simulink model "Adaptive_Cruise_Contro_Final_KD_JB_TV_22"  (R2020a)
settings: Solver=FixedStepAuto  StartTime=0.0  StopTime=10.0  RelTol=1e-3  EnableMultiTasking=on
libraries: arduinolib x14, arduinosensorlib x1
settings Model: SILPILModeSetting=veronly  ExtModeTrigDuration=2  Creator=anuru  LastModifiedBy=anuru
settings OptimizationCC: EnhancedBackFolding=on  PassReuseOutputArgsAs=Individual arguments  ZeroExternalMemoryAtStartup=off  ZeroInternalMemoryAtStartup=off  MaxStackSize=64  OptimizeBlockOrder=speed  DifferentSizesBufferReuse=on  OptimizationCustomize=off  EfficientTunableParamExpr=on
settings DebuggingCC: ParameterTunabilityLossMsg=error
settings HardwareCC: ProdBitPerInt=16  ProdBitPerPointer=16  ProdBitPerSizeT=16  ProdBitPerPtrDiffT=16  ProdLargestAtomicFloat=None  ProdWordSize=8  ProdHWDeviceType=Atmel->AVR
settings SFSimCC: MATLABDynamicMemAlloc=off
settings RTWCC: SystemTargetFile=ert.tlc  HardwareBoard=Arduino Uno  TLCOptions=-aInlineSetEventsForThisBaseRateFcn=TLC_FALSE -aSuppressMultiTaskScheduler=TLC_FALSE -aRateBasedStepFcn=1  TemplateMakefile=ert_default_tmf  Toolchain=Arduino AVR  BuildConfiguration=Faster Runs
settings CodeAppCC: ForceParamTrailComments=on  IgnoreCustomStorageClasses=off  OperatorAnnotations=on  SimulinkDataObjDesc=on  SFDataObjDesc=on  InsertBlockDesc=on
settings ERTTargetCC: SupportContinuousTime=on  SupportVariableSizeSignals=on  ExtModeStaticAllocSize=250

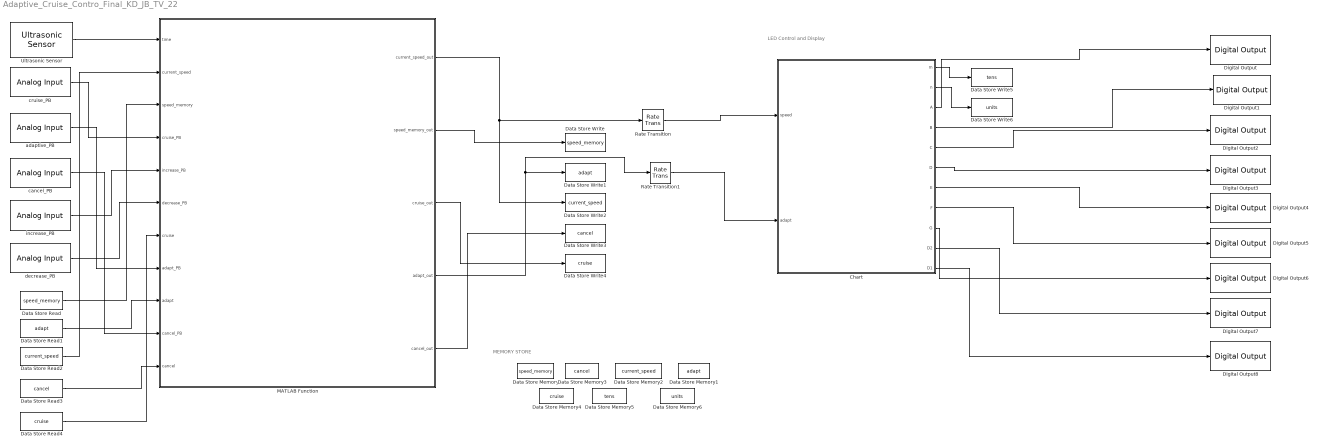
== system Adaptive_Cruise_Contro_Final_KD_JB_TV_22 ==
  note: MEMORY STORE
  note: LED Control and Display
  Chart : Stateflow chart  TreatAsAtomicUnit=on  SystemSampleTime=0.001
      settings: PortSchema="{\"entries\":[{\"content\":{\"sides\":[{\"content\":{\"connectorIds\":[\"In1\",\"In2\"]},\"type\":\"ConnectorPlacement.EquallySpacedRectSide\",\"uuid\":\"44d2400a-07fc-4d50-ac25-34b2e5b65562\"},{\"content\":{\"connectorIds\":[\"Out10\",\"Out11\",\"Out1\",\"Out2\",\"Out3\",\"Out4\",\"Out5\",\"Out6\",\"Out7\",\"Out9\",\"Out8\"],\"side\":\"RIGHT\"},\"type\":\"ConnectorPlacement.EquallySpacedRectSide\",\"uuid\":\"b0f8c742-c813-41dd-9ffd-889c5ddd76f2\"},{\"content\":{\"connectorIds\":[],\"side\":\"TOP\"},\"type\":\"ConnectorPlacement.EquallySpacedRectSide\",\"uuid\":\"01dd0f2c-e697-4f0c-a19d-ad69aab25abe\"}]},\"type\":\"ConnectorPlacement.EquallySpacedConnector\",\"uuid\":\"9d4b280d-d5e4-4ff2-9163-760fba15e8f7\"}],\"packageUris\":[\"http://schema.mathworks.com/mf0/Connector/19700101\"],\"version\":\"1.0\"}"
  Data Store Memory : DataStoreMemory  DataStoreName=speed_memory  ReadBeforeWriteMsg=warning  WriteAfterWriteMsg=warning  WriteAfterReadMsg=warning  ShowAdditionalParam=off
  Data Store Memory1 : DataStoreMemory  DataStoreName=adapt  ReadBeforeWriteMsg=warning  WriteAfterWriteMsg=warning  WriteAfterReadMsg=warning  ShowAdditionalParam=off
  Data Store Memory2 : DataStoreMemory  DataStoreName=current_speed  ReadBeforeWriteMsg=warning  WriteAfterWriteMsg=warning  WriteAfterReadMsg=warning  ShowAdditionalParam=off
  Data Store Memory3 : DataStoreMemory  DataStoreName=cancel  ReadBeforeWriteMsg=warning  WriteAfterWriteMsg=warning  WriteAfterReadMsg=warning  ShowAdditionalParam=off
  Data Store Memory4 : DataStoreMemory  DataStoreName=cruise  ReadBeforeWriteMsg=warning  WriteAfterWriteMsg=warning  WriteAfterReadMsg=warning  ShowAdditionalParam=off
  Data Store Memory5 : DataStoreMemory  DataStoreName=tens  ReadBeforeWriteMsg=warning  WriteAfterWriteMsg=warning  WriteAfterReadMsg=warning  ShowAdditionalParam=off
  Data Store Memory6 : DataStoreMemory  DataStoreName=units  ReadBeforeWriteMsg=warning  WriteAfterWriteMsg=warning  WriteAfterReadMsg=warning  ShowAdditionalParam=off
  Data Store Read : DataStoreRead  DataStoreName=speed_memory
  Data Store Read1 : DataStoreRead  DataStoreName=adapt
  Data Store Read2 : DataStoreRead  DataStoreName=current_speed
  Data Store Read3 : DataStoreRead  DataStoreName=cancel
  Data Store Read4 : DataStoreRead  DataStoreName=cruise
  Data Store Write : DataStoreWrite  DataStoreName=speed_memory
  Data Store Write1 : DataStoreWrite  DataStoreName=adapt
  Data Store Write2 : DataStoreWrite  DataStoreName=current_speed
  Data Store Write3 : DataStoreWrite  DataStoreName=cancel
  Data Store Write4 : DataStoreWrite  DataStoreName=cruise
  Data Store Write5 : DataStoreWrite  DataStoreName=tens
  Data Store Write6 : DataStoreWrite  DataStoreName=units
  Digital Output : arduinolib/Digital Output  pinNumber=2  Direction=output  blockPlatform=arduino
  Digital Output1 : arduinolib/Digital Output  pinNumber=3  Direction=output  blockPlatform=arduino
  Digital Output2 : arduinolib/Digital Output  pinNumber=4  Direction=output  blockPlatform=arduino
  Digital Output3 : arduinolib/Digital Output  pinNumber=5  Direction=output  blockPlatform=arduino
  Digital Output4 : arduinolib/Digital Output  pinNumber=6  Direction=output  blockPlatform=arduino
  Digital Output5 : arduinolib/Digital Output  pinNumber=7  Direction=output  blockPlatform=arduino
  Digital Output6 : arduinolib/Digital Output  pinNumber=8  Direction=output  blockPlatform=arduino
  Digital Output7 : arduinolib/Digital Output  pinNumber=9  Direction=output  blockPlatform=arduino
  Digital Output8 : arduinolib/Digital Output  pinNumber=10  Direction=output  blockPlatform=arduino
  MATLAB Function : MATLAB Function  TreatAsAtomicUnit=on  SystemSampleTime=0.3
  Rate Transition : RateTransition  Deterministic=off  OutPortSampleTime=0.001
  Rate Transition1 : RateTransition  Deterministic=off  OutPortSampleTime=0.001
  Ultrasonic Sensor : arduinosensorlib/Ultrasonic Sensor  NumSignalPins=2  TrigPin=11  EchoPin=12  SignalPin=3  SampleTime_=0.3  blockPlatform=ARDUINO
      settings: SourceProductBaseCode=ARDUINO
  adaptive_PB : arduinolib/Analog Input  pinNumber=3  ReadResultsOnly=off  ConversionTriggerSource=Software  ExternalTriggerType=uint32( 0 )  OutputDataType=uint16  EnableConversionCompleteNotify=off  EnableOuputStatus=off  SampleTime=-1  blockPlatform=arduino
  cancel_PB : arduinolib/Analog Input  pinNumber=2  ReadResultsOnly=off  ConversionTriggerSource=Software  ExternalTriggerType=uint32( 0 )  OutputDataType=uint16  EnableConversionCompleteNotify=off  EnableOuputStatus=off  SampleTime=-1  blockPlatform=arduino
  cruise_PB : arduinolib/Analog Input  pinNumber=5  ReadResultsOnly=off  ConversionTriggerSource=Software  ExternalTriggerType=uint32( 0 )  OutputDataType=uint16  EnableConversionCompleteNotify=off  EnableOuputStatus=off  SampleTime=-1  blockPlatform=arduino
  decrease_PB : arduinolib/Analog Input  pinNumber=0  ReadResultsOnly=off  ConversionTriggerSource=Software  ExternalTriggerType=uint32( 0 )  OutputDataType=uint16  EnableConversionCompleteNotify=off  EnableOuputStatus=off  SampleTime=-1  blockPlatform=arduino
  increase_PB : arduinolib/Analog Input  pinNumber=1  ReadResultsOnly=off  ConversionTriggerSource=Software  ExternalTriggerType=uint32( 0 )  OutputDataType=uint16  EnableConversionCompleteNotify=off  EnableOuputStatus=off  SampleTime=-1  blockPlatform=arduino
  wires:
  Chart/1(A) -> Digital Output/1
  Chart/2(B) -> Digital Output1/1
  Chart/3(C) -> Digital Output2/1
  Chart/4(D) -> Digital Output3/1
  Chart/5(E) -> Digital Output4/1
  Chart/6(F) -> Digital Output5/1
  Chart/7(G) -> Digital Output6/1
  Chart/9(D2) -> Digital Output7/1
  Chart/8(D1) -> Digital Output8/1
  Chart/10(m) -> Data Store Write5/1
  Chart/11(n) -> Data Store Write6/1
  Data Store Read2/1 -> MATLAB Function/2(current_speed)
  Data Store Read/1 -> MATLAB Function/3(speed_memory)
  Data Store Read3/1 -> MATLAB Function/11(cancel)
  Data Store Read4/1 -> MATLAB Function/7(cruise)
  Data Store Read1/1 -> MATLAB Function/9(adapt)
  decrease_PB/1 -> MATLAB Function/6(decrease_PB)
  increase_PB/1 -> MATLAB Function/5(increase_PB)
  cancel_PB/1 -> MATLAB Function/10(cancel_PB)
  adaptive_PB/1 -> MATLAB Function/8(adapt_PB)
  cruise_PB/1 -> MATLAB Function/4(cruise_PB)
  MATLAB Function/1(current_speed_out) -> Rate Transition/1, Data Store Write2/1
  MATLAB Function/2(speed_memory_out) -> Data Store Write/1
  MATLAB Function/3(cruise_out) -> Data Store Write4/1
  MATLAB Function/4(adapt_out) -> Rate Transition1/1, Data Store Write1/1
  MATLAB Function/5(cancel_out) -> Data Store Write3/1
  Rate Transition/1 -> Chart/1(speed)
  Rate Transition1/1 -> Chart/2(adapt)
  Ultrasonic Sensor/1 -> MATLAB Function/1(time)

== matlab function Adaptive_Cruise_Contro_Final_KD_JB_TV_22/MATLAB Function ==
  data: time input; current_speed_out output; current_speed input; speed_memory input; cruise_PB input; increase_PB input; decrease_PB input; cruise input; adapt_PB input; adapt input; cancel_PB input; cancel input; speed_memory_out output; cruise_out output; adapt_out output; cancel_out output
% Adaptive Cruise Control using Arduino with Simulink
% Group 22
% 12th of August 2020
% Kurukulasuriya Dias, Jiten Bhatt, Tejaswini Vekaria
% GENG8030-2-R-2020S
% Professor Roozbeh Razavi Far
%-----NOTE----%
%PB's cruise,adapt,cancel,accelerate and decelerate are set in analog pins
%analog pins A5,A3,A2,A1,A0 respectively
function [current_speed_out, speed_memory_out,cruise_out, adapt_out, cancel_out] = logic_control(time,current_speed,speed_memory,cruise_PB,increase_PB, decrease_PB,cruise,adapt_PB,adapt,cancel_PB,cancel)
% Check for Set Cruise PB, Adapt PB and Cancel PB is pressed and set
% relevant output for next step of the function
% Analog voltage converted to digital value 0-1023 for Arduino Uno Board
% takes in speed to memory
if (cruise_PB>200)
    speed_memory_out=current_speed;
    cruise_out=1;
    adapt_out=0;
    cancel_out=cancel;
elseif (adapt_PB>200)
    speed_memory_out=current_speed;
    adapt_out=1;
    cruise_out=0;
    cancel_out=0;
elseif (cancel_PB>200)
    speed_memory_out=speed_memory;
    cancel_out=1;
    cruise_out=0;
    adapt_out=0;  
else
    speed_memory_out=speed_memory;
    cruise_out=cruise;
    adapt_out=adapt;
    cancel_out=cancel;
end
%when cruise, adapt, cancel, increase and decrease PBs are pressed, code 
%for speed control and adaptive settings and cancel cruise and adaptive
%when in cruise mode checks if increase or decrease PB's are pressed and
%speed is changed accordingly otherwise stays constant
if (cruise==1)
    if (increase_PB>200)&&(adapt==0)
        current_speed_out=current_speed+1;
        speed_memory_out = current_speed;
    elseif (decrease_PB>200)&&(adapt==0)&&(current_speed>0)
        current_speed_out = current_speed-1;
        speed_memory_out = current_speed;
    else
        speed_memory_out = speed_memory;
        current_speed_out = current_speed;
    end
%When in adaptive mode check position from other car and if less than or
%equalto 15 the speed slows or if further away speeds up to memory speed
%and stays constant
elseif (adapt==1)
    position=(time*343)/2;
    if (position<=15)&&(current_speed>0)
        current_speed_out=current_speed-1;
    else
        if (speed_memory>=1)
            if (current_speed>speed_memory)&&(current_speed>0)
                current_speed_out=current_speed-1;
            elseif (current_speed<speed_memory)
                if(position>15)
                    current_speed_out=current_speed+1;
                else
                    current_speed_out=current_speed;
                end
            else
                current_speed_out=current_speed;
            end
        else
            current_speed_out=current_speed;
        end
    end
%When cancel is pressed, gets out of adaptive or cruise mode, speed
%decreases over time
elseif (cancel==1)
    if current_speed>0
        current_speed_out=current_speed-1;
    else
        current_speed_out=current_speed;
        cancel_out=0;
    end
%Increase PB pressed, increases speed
elseif(increase_PB>200)&&(adapt==0)
    current_speed_out = current_speed+1;
% Decrease PB pressed decreases speed
elseif(decrease_PB>200)&&(adapt==0)&&(current_speed>0)
    current_speed_out = current_speed-1;
% When no PBs are pressed, speed decreases
else
    if(current_speed>0)
        current_speed_out = current_speed-1;
    else
        current_speed_out = current_speed;
    end
end
end

== stateflow chart Adaptive_Cruise_Contro_Final_KD_JB_TV_22/Chart ==
  state CALCULATION
    entry:
    m=floor(speed/10);
    n=speed-(m*10);
  state CONTROL_OUTPUT
  state NonAdaptive
  state Adaptive
  state GREATER_THAN_99
    entry:
    D1=0;
    D2=1;
    A=1;B=1;C=1;D=1;E=1;F=1;G=0;
  state DISPLAY5
    entry:
    D1=1;
    D2=0;
    A=1;B=0;C=1;D=1;E=0;F=1;G=1;
  state DISPLAY6
    entry:
    D1=1;
    D2=0;
    A=1;B=0;C=1;D=1;E=1;F=1;G=1;
  state DISPLAY8
    entry:
    D1=1;
    D2=0;
    A=1;B=1;C=1;D=1;E=1;F=1;G=1;
  state DISPLAY7
    entry:
    D1=1;
    D2=0;
    A=1;B=1;C=1;D=0;E=0;F=0;G=0;
  state DISPLAY4
    entry:
    D1=1;
    D2=0;
    A=0;B=1;C=1;D=0;E=0;F=1;G=1;
  state DISPLAY9
    entry:
    D1=1;
    D2=0;
    A=1;B=1;C=1;D=1;E=0;F=1;G=1;
  state DISPLAY1
    entry:
    D1=1;
    D2=0;
    A=0;B=1;C=1;D=0;E=0;F=0;G=0;
  state DISPLAY2
    entry:
    D1=1;
    D2=0;
    A=1;B=1;C=0;D=1;E=1;F=0;G=1;
  state DISPLAY0
    entry:
    D1=1;
    D2=0;
    A=1;B=1;C=1;D=1;E=1;F=1;G=0;
  state DISPLAY3
    entry:
    D1=1;
    D2=0;
    A=1;B=1;C=1;D=1;E=0;F=0;G=1;
  state CONTROL3
  state DISPLAY00
    entry:
    D1=0;
    D2=1;
    A=1;B=1;C=1;D=1;E=1;F=1;G=0;
  state DISPLAY11
    entry:
    D1=0;
    D2=1;
    A=0;B=1;C=1;D=0;E=0;F=0;G=0;
  state DISPLAY22
    entry:
    D1=0;
    D2=1;
    A=1;B=1;C=0;D=1;E=1;F=0;G=1;
  state DISPLAY33
    entry:
    D1=0;
    D2=1;
    A=1;B=1;C=1;D=1;E=0;F=0;G=1;
  state Adapt
  state DISPLAY44
    entry:
    D1=0;
    D2=1;
    A=0;B=1;C=1;D=0;E=0;F=1;G=1;
  state CONTROL2
  state NonAdapt
  state DISPLAY55
    entry:
    D1=0;
    D2=1;
    A=1;B=0;C=1;D=1;E=0;F=1;G=1;
  state DISPLAY66
    entry:
    D1=0;
    D2=1;
    A=1;B=0;C=1;D=1;E=1;F=1;G=1;
  state DISPLAY77
    entry:
    D1=0;
    D2=1;
    A=1;B=1;C=1;D=0;E=0;F=0;G=0;
  state DISPLAY88
    entry:
    D1=0;
    D2=1;
    A=1;B=1;C=1;D=1;E=1;F=1;G=1;
  state DISPLAY99
    entry:
    D1=0;
    D2=1;
    A=1;B=1;C=1;D=1;E=0;F=1;G=1;
  (default) -> CALCULATION
  Adaptive -> CALCULATION : after(20,msec)
  NonAdaptive -> CALCULATION
  CALCULATION -> CONTROL_OUTPUT : after(2,msec)
  CONTROL_OUTPUT -> DISPLAY1 [order 4] : [m==1]
  CONTROL_OUTPUT -> DISPLAY0 [order 5] : [m==0]
  CONTROL_OUTPUT -> DISPLAY2 [order 3] : [m==2]
  CONTROL_OUTPUT -> DISPLAY3 [order 1] : [m==3]
  CONTROL_OUTPUT -> DISPLAY4 [order 6] : [m==4]
  CONTROL_OUTPUT -> DISPLAY5 [order 2] : [m==5]
  CONTROL_OUTPUT -> DISPLAY6 [order 7] : [m==6]
  CONTROL_OUTPUT -> DISPLAY7 [order 8] : [m==7]
  CONTROL_OUTPUT -> DISPLAY8 [order 9] : [m==8]
  CONTROL_OUTPUT -> DISPLAY9 [order 10] : [m==9]
  CONTROL_OUTPUT -> GREATER_THAN_99 [order 11] : [speed>99||speed<0]
  (junction 138) -> NonAdaptive [order 2] : [adapt==0]
  (junction 138) -> Adaptive [order 1] : [adapt==1]
  DISPLAY7 -> CONTROL3
  DISPLAY8 -> CONTROL3
  DISPLAY6 -> CONTROL3
  DISPLAY4 -> CONTROL3
  DISPLAY2 -> CONTROL3
  DISPLAY5 -> CONTROL3
  DISPLAY9 -> CONTROL3
  GREATER_THAN_99 -> CONTROL3
  DISPLAY3 -> CONTROL3
  DISPLAY0 -> CONTROL3
  DISPLAY1 -> CONTROL3
  CONTROL2 -> DISPLAY00 [order 1] : [n==0]
  DISPLAY00 -> (junction 138)
  CONTROL2 -> DISPLAY11 [order 4] : [n==1]
  DISPLAY11 -> (junction 138)
  CONTROL3 -> NonAdapt [order 2] : [adapt==0]
  CONTROL3 -> Adapt [order 1] : [adapt==1]
  DISPLAY22 -> (junction 138)
  CONTROL2 -> DISPLAY44 [order 2] : [n==4]
  CONTROL2 -> DISPLAY22 [order 5] : [n==2]
  Adapt -> CONTROL2 : after(20,msec)
  DISPLAY33 -> (junction 138)
  CONTROL2 -> DISPLAY33 [order 6] : [n==3]
  CONTROL2 -> DISPLAY55 [order 7] : [n==5]
  DISPLAY99 -> (junction 138)
  DISPLAY77 -> (junction 138)
  DISPLAY55 -> (junction 138)
  DISPLAY66 -> (junction 138)
  DISPLAY44 -> (junction 138)
  DISPLAY88 -> (junction 138)
  NonAdapt -> CONTROL2 : after(2,msec)
  CONTROL2 -> DISPLAY66 [order 9] : [n==6]
  CONTROL2 -> DISPLAY77 [order 8] : [n==7]
  CONTROL2 -> DISPLAY88 [order 10] : [n==8]
  CONTROL2 -> DISPLAY99 [order 3] : [n==9]
  data: speed input; A output; B output; C output; D output; E output; F output; G output; D1 output; D2 output; m output; n output; adapt input
